simulink model "reportsim"  (R2022a)
settings: Solver=VariableStepAuto  StartTime=0.0  StopTime=50  RelTol=1e-7
undefined symbols (not defined in the file): c1, c2, k1, k2, m1, m2
settings Model: Creator=sucho  LastModifiedBy=sucho
settings SolverCC: MaxConsecutiveMinStep=2

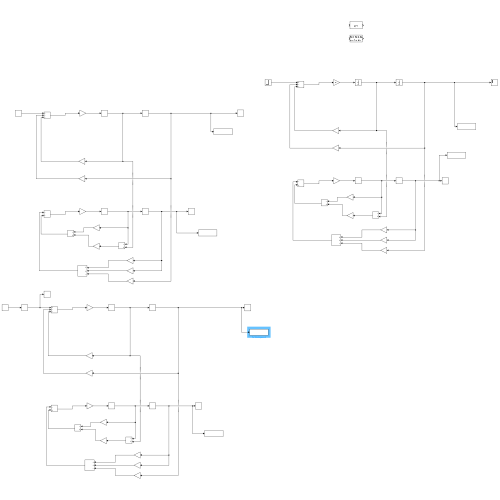
[thumbnail: Simulink's stored preview of the top-level diagram]
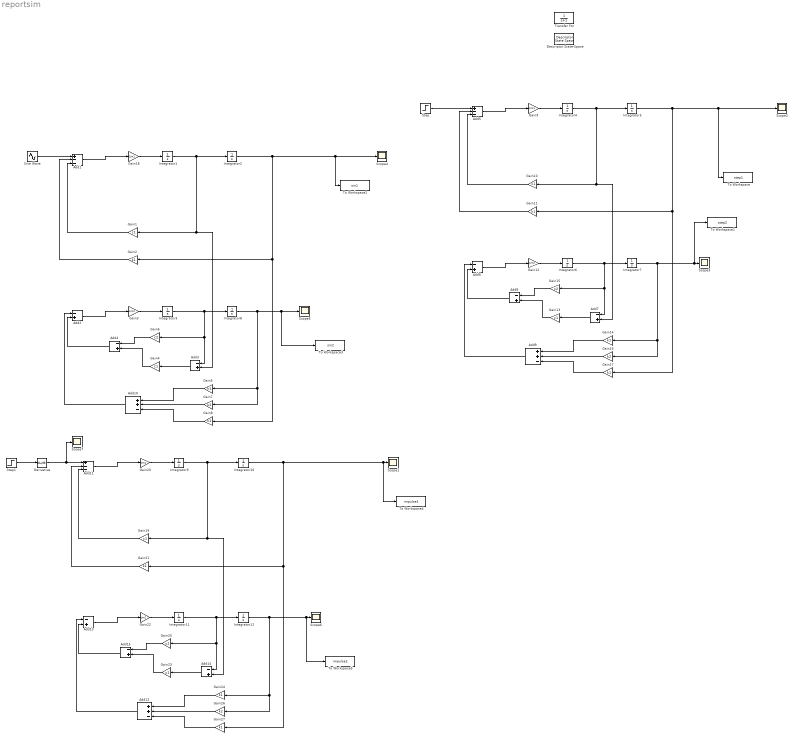
== system reportsim ==
  Add1 : Sum  Inputs=+--
  Add10 : Sum  Inputs=++-
  Add11 : Sum  Inputs=+--
  Add12 : Sum  Inputs=++-
  Add{2..4,6..8,13..15} (9 alike) : Sum  Inputs=-+
  Add5 : Sum  Inputs=+--
  Add9 : Sum  Inputs=++-
  Derivative : Derivative
  Descriptor State-Space : DescriptorStateSpace
  Gain{1,4,10,13,19,23} (6 alike) : Gain  Gain=c1
  Gain{2,5,8,11,14,17,21,24,27} (9 alike) : Gain  Gain=k1
  Gain12 : Gain  Gain=1/m2
  Gain15 : Gain  Gain=c2
  Gain16 : Gain  Gain=k2
  Gain18 : Gain  Gain=2/m1
  Gain20 : Gain  Gain=2/m1
  Gain22 : Gain  Gain=1/m2
  Gain25 : Gain  Gain=c2
  Gain26 : Gain  Gain=k2
  Gain3 : Gain  Gain=1/m2
  Gain6 : Gain  Gain=c2
  Gain7 : Gain  Gain=k2
  Gain9 : Gain  Gain=1/m1
  Integrator{1..2,4..5,9..10} (6 alike) : Integrator  InitialCondition=1
  Integrator{3,6..8,11..12} (6 alike) : Integrator
  Scope{1..7} (7 alike) : Scope
  Sine Wave : Sin  SampleTime=0
  Step : Step  Time=0  SampleTime=0
  Step1 : Step  SampleTime=0
  To Workspace : ToWorkspace  VariableName=step1  SaveFormat=Timeseries  SampleTime=-1
  To Workspace1 : ToWorkspace  VariableName=step2  SaveFormat=Timeseries  SampleTime=-1
  To Workspace2 : ToWorkspace  VariableName=sin1  SaveFormat=Timeseries  SampleTime=-1
  To Workspace3 : ToWorkspace  VariableName=sin2  SaveFormat=Timeseries  SampleTime=-1
  To Workspace4 : ToWorkspace  VariableName=impulse1  SaveFormat=Timeseries  SampleTime=-1
  To Workspace5 : ToWorkspace  VariableName=impulse2  SaveFormat=Timeseries  SampleTime=-1
  Transfer Fcn : TransferFcn  Denominator=[1 1]
  wires:
  Gain17/1 -> Add9/3
  Gain16/1 -> Add9/2
  Add7/1 -> Gain13/1
  Add8/1 -> Add6/2
  Add6/1 -> Gain12/1
  Integrator7/1 -> To Workspace1/1, Scope3/1, Gain16/1, Gain14/1
  Gain12/1 -> Integrator6/1
  Add9/1 -> Add6/1
  Add5/1 -> Gain9/1
  Gain9/1 -> Integrator4/1
  Integrator6/1 -> Add7/1, Gain15/1, Integrator7/1
  Gain15/1 -> Add8/1
  Step/1 -> Add5/1
  Gain13/1 -> Add8/2
  Gain11/1 -> Add5/2
  Gain10/1 -> Add5/3
  Gain14/1 -> Add9/1
  Integrator5/1 -> To Workspace/1, Scope2/1, Gain17/1, Gain11/1
  Integrator4/1 -> Add7/2, Gain10/1, Integrator5/1
  Integrator1/1 -> Add3/2, Gain1/1, Integrator2/1
  Gain5/1 -> Add10/1
  Integrator3/1 -> Add3/1, Gain6/1, Integrator8/1
  Gain8/1 -> Add10/3
  Integrator2/1 -> To Workspace2/1, Scope4/1, Gain8/1, Gain2/1
  Gain4/1 -> Add4/2
  Add2/1 -> Gain3/1
  Gain2/1 -> Add1/2
  Add1/1 -> Gain18/1
  Gain3/1 -> Integrator3/1
  Add4/1 -> Add2/2
  Gain1/1 -> Add1/3
  Gain6/1 -> Add4/1
  Gain18/1 -> Integrator1/1
  Add10/1 -> Add2/1
  Add3/1 -> Gain4/1
  Integrator8/1 -> To Workspace3/1, Scope5/1, Gain7/1, Gain5/1
  Gain7/1 -> Add10/2
  Sine Wave/1 -> Add1/1
  Integrator11/1 -> Add14/1, Gain25/1, Integrator12/1
  Derivative/1 -> Scope7/1, Add11/1
  Gain19/1 -> Add11/3
  Gain24/1 -> Add12/1
  Gain22/1 -> Integrator11/1
  Gain20/1 -> Integrator9/1
  Gain25/1 -> Add15/1
  Add12/1 -> Add13/1
  Add14/1 -> Gain23/1
  Gain26/1 -> Add12/2
  Gain27/1 -> Add12/3
  Integrator12/1 -> To Workspace5/1, Scope6/1, Gain26/1, Gain24/1
  Gain23/1 -> Add15/2
  Add11/1 -> Gain20/1
  Integrator10/1 -> To Workspace4/1, Scope1/1, Gain27/1, Gain21/1
  Integrator9/1 -> Add14/2, Gain19/1, Integrator10/1
  Add13/1 -> Gain22/1
  Gain21/1 -> Add11/2
  Add15/1 -> Add13/2
  Step1/1 -> Derivative/1
